simulink model "real_pid_implementation"  (R2025b)
settings: Solver=VariableStepAuto  StartTime=0.0  StopTime=10.0  RelTol=1e-3
settings Model: Creator=PROBOOK  LastModifiedBy=PROBOOK

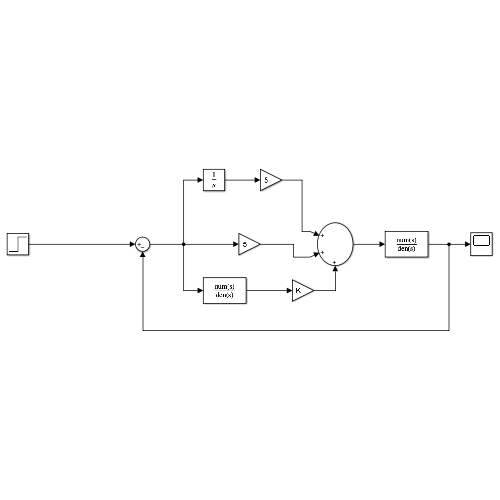
[thumbnail: Simulink's stored preview of the top-level diagram]
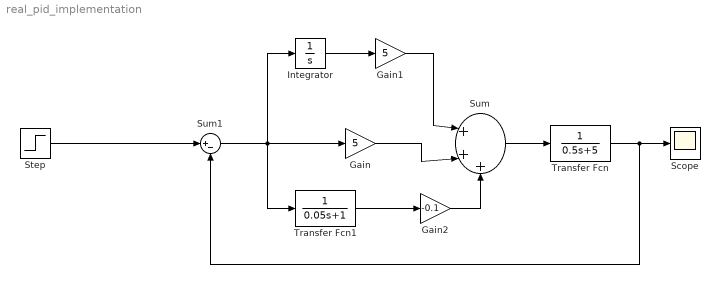
== system real_pid_implementation ==
  Gain : Gain  Gain=5
  Gain1 : Gain  Gain=5
  Gain2 : Gain  Gain=-0.1
  Integrator : Integrator
  Scope : Scope
      settings: ActiveDisplayYMinimum=-1.1211023745217916  ActiveDisplayYMaximum=10.089921370696127
  Step : Step  Before=6  After=9  SampleTime=0
  Sum : Sum  Inputs=|+++
  Sum1 : Sum  Inputs=|+-
  Transfer Fcn : TransferFcn  Denominator=[0.5 5]
  Transfer Fcn1 : TransferFcn  Denominator=[0.05 1]
  wires:
  Step/1 -> Sum1/1
  Sum1/1 -> Transfer Fcn1/1, Integrator/1, Gain/1
  Integrator/1 -> Gain1/1
  Gain/1 -> Sum/2
  Gain1/1 -> Sum/1
  Gain2/1 -> Sum/3
  Sum/1 -> Transfer Fcn/1
  Transfer Fcn/1 -> Sum1/2, Scope/1
  Transfer Fcn1/1 -> Gain2/1
